simulink model "tanques_inter"  (R2020b)
settings: Solver=VariableStepAuto  StartTime=0.0  StopTime=10.0  RelTol=1e-3
values from neighbouring files (symbols this model uses):
  C1 = 40    [tanques_interconectados.m]
  C2 = 60    [tanques_interconectados.m]
  R1 = 10    [tanques_interconectados.m]
  R2 = 28    [tanques_interconectados.m]
settings Model: Creator=carma  LastModifiedBy=carma

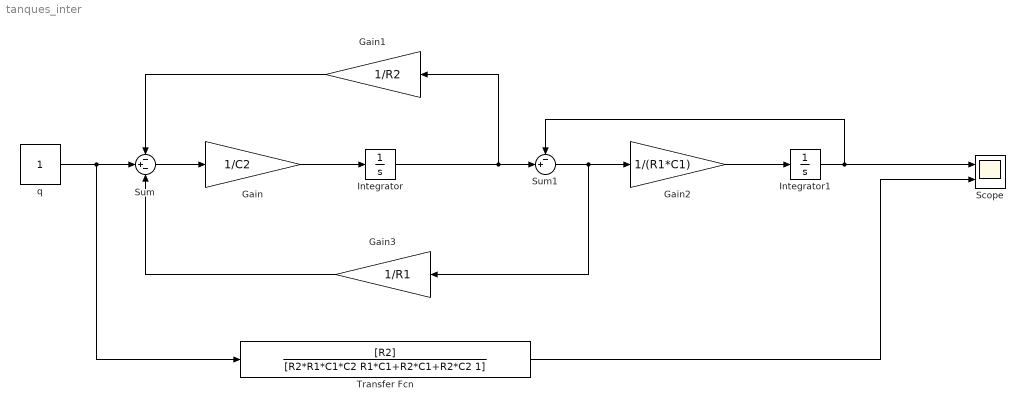
== system tanques_inter ==
  Gain : Gain  Gain=1/C2
  Gain1 : Gain  Gain=1/R2
  Gain2 : Gain  Gain=1/(R1*C1)
  Gain3 : Gain  Gain=1/R1
  Integrator : Integrator
  Integrator1 : Integrator
  Scope : Scope  NumInputPorts=2
  Sum : Sum  Inputs=-+-
  Sum1 : Sum  Inputs=-+|
  Transfer Fcn : TransferFcn  Numerator=[R2]  Denominator=[R2*R1*C1*C2 R1*C1+R2*C1+R2*C2 1]
  q : Constant  VectorParams1D=off  SampleTime=-1
  wires:
  q/1 -> Transfer Fcn/1, Sum/2
  Gain3/1 -> Sum/3
  Sum/1 -> Gain/1
  Gain/1 -> Integrator/1
  Integrator/1 -> Gain1/1, Sum1/2
  Gain1/1 -> Sum/1
  Gain2/1 -> Integrator1/1
  Integrator1/1 -> Sum1/1, Scope/1
  Sum1/1 -> Gain3/1, Gain2/1
  Transfer Fcn/1 -> Scope/2
